simulink model "Full_Charge"  (R2020a)
settings: Solver=VariableStepAuto  StartTime=0.0  StopTime=45*60*60  RelTol=1e-3
values from neighbouring files (symbols this model uses):
  BlySyreON = 1    [sim_starter.m]
  CurrentChargeBlySyre = load    [sim_starter.m]
  CurrentChargeLiLille = load    [sim_starter.m]
  CurrentChargeLiStor = load    [sim_starter.m]
  CurrentChargeNiMH = load    [sim_starter.m]
  CurrentChargeSaltVand = load    [sim_starter.m]
  LiIonLilleON = 1    [sim_starter.m]
  LiIonStorON = 1    [sim_starter.m]
  NiMHON = 1    [sim_starter.m]
  SaltVandON = 1    [sim_starter.m]
  SwitchCurrentBlySyre = 1    [sim_starter.m]
  SwitchCurrentLiLille = 1    [sim_starter.m]
  SwitchCurrentLiStor = 1    [sim_starter.m]
  SwitchCurrentNiMH = 1    [sim_starter.m]
  SwitchCurrentSaltVand = 1    [sim_starter.m]
  VoltageChargeBlySyre = 0    [sim_starter.m]
  VoltageChargeLiLille = load    [sim_starter.m]
  VoltageChargeLiStor = load    [sim_starter.m]
  VoltageChargeNiMH = load    [sim_starter.m]
  VoltageChargeSaltVand = load    [sim_starter.m]
undefined symbols (not defined in the file or in its folder): Hydride, Metal, Nickel
libraries: nesl_utility x37, fl_lib x35, ee_lib x8, powerlib x7, electricdrivelib x1
(part 1 of 2)
settings Model: Creator=phili  LastModifiedBy=jenslawl

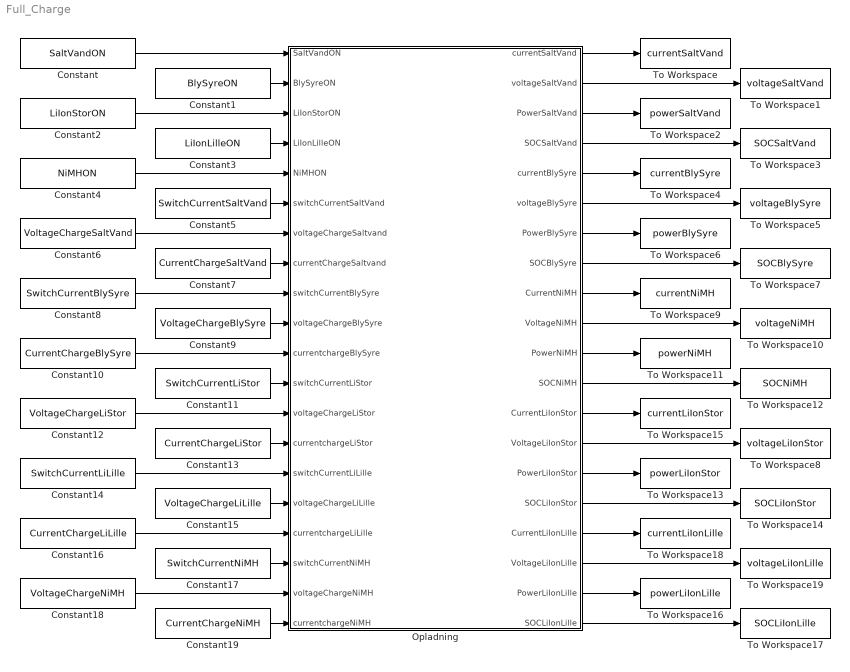
== system Full_Charge ==
  Constant : Constant  Value=SaltVandON
  Constant1 : Constant  Value=BlySyreON
  Constant10 : Constant  Value=CurrentChargeBlySyre
  Constant11 : Constant  Value=SwitchCurrentLiStor
  Constant12 : Constant  Value=VoltageChargeLiStor
  Constant13 : Constant  Value=CurrentChargeLiStor
  Constant14 : Constant  Value=SwitchCurrentLiLille
  Constant15 : Constant  Value=VoltageChargeLiLille
  Constant16 : Constant  Value=CurrentChargeLiLille
  Constant17 : Constant  Value=SwitchCurrentNiMH
  Constant18 : Constant  Value=VoltageChargeNiMH
  Constant19 : Constant  Value=CurrentChargeNiMH
  Constant2 : Constant  Value=LiIonStorON
  Constant3 : Constant  Value=LiIonLilleON
  Constant4 : Constant  Value=NiMHON
  Constant5 : Constant  Value=SwitchCurrentSaltVand
  Constant6 : Constant  Value=VoltageChargeSaltVand
  Constant7 : Constant  Value=CurrentChargeSaltVand
  Constant8 : Constant  Value=SwitchCurrentBlySyre
  Constant9 : Constant  Value=VoltageChargeBlySyre
  Opladning : Subsystem
  To Workspace : ToWorkspace  VariableName=currentSaltVand  SampleTime=-1
  To Workspace1 : ToWorkspace  VariableName=voltageSaltVand  SampleTime=-1
  To Workspace10 : ToWorkspace  VariableName=voltageNiMH  SampleTime=-1
  To Workspace11 : ToWorkspace  VariableName=powerNiMH  SampleTime=-1
  To Workspace12 : ToWorkspace  VariableName=SOCNiMH  SampleTime=-1
  To Workspace13 : ToWorkspace  VariableName=powerLiIonStor  SampleTime=-1
  To Workspace14 : ToWorkspace  VariableName=SOCLiIonStor  SampleTime=-1
  To Workspace15 : ToWorkspace  VariableName=currentLiIonStor  SampleTime=-1
  To Workspace16 : ToWorkspace  VariableName=powerLiIonLille  SampleTime=-1
  To Workspace17 : ToWorkspace  VariableName=SOCLiIonLille  SampleTime=-1
  To Workspace18 : ToWorkspace  VariableName=currentLiIonLille  SampleTime=-1
  To Workspace19 : ToWorkspace  VariableName=voltageLiIonLille  SampleTime=-1
  To Workspace2 : ToWorkspace  VariableName=powerSaltVand  SampleTime=-1
  To Workspace3 : ToWorkspace  VariableName=SOCSaltVand  SampleTime=-1
  To Workspace4 : ToWorkspace  VariableName=currentBlySyre  SampleTime=-1
  To Workspace5 : ToWorkspace  VariableName=voltageBlySyre  SampleTime=-1
  To Workspace6 : ToWorkspace  VariableName=powerBlySyre  SampleTime=-1
  To Workspace7 : ToWorkspace  VariableName=SOCBlySyre  SampleTime=-1
  To Workspace8 : ToWorkspace  VariableName=voltageLiIonStor  SampleTime=-1
  To Workspace9 : ToWorkspace  VariableName=currentNiMH  SampleTime=-1
  wires:
  Constant/1 -> Opladning/1(SaltVandON)
  Constant1/1 -> Opladning/2(BlySyreON)
  Constant2/1 -> Opladning/3(LiIonStorON)
  Constant3/1 -> Opladning/4(LiIonLilleON)
  Constant4/1 -> Opladning/5(NiMHON)
  Constant5/1 -> Opladning/6(switchCurrentSaltVand)
  Constant6/1 -> Opladning/7(voltageChargeSaltvand)
  Constant7/1 -> Opladning/8(currentChargeSaltvand)
  Constant8/1 -> Opladning/9(switchCurrentBlySyre)
  Constant9/1 -> Opladning/10(voltageChargeBlySyre)
  Constant10/1 -> Opladning/11(currentchargeBlySyre)
  Constant11/1 -> Opladning/12(switchCurrentLiStor)
  Constant12/1 -> Opladning/13(voltageChargeLiStor)
  Constant13/1 -> Opladning/14(currentchargeLiStor)
  Constant14/1 -> Opladning/15(switchCurrentLiLille)
  Constant15/1 -> Opladning/16(voltageChargeLiLille)
  Constant16/1 -> Opladning/17(currentchargeLiLille)
  Constant17/1 -> Opladning/18(switchCurrentNiMH)
  Constant18/1 -> Opladning/19(voltageChargeNiMH)
  Constant19/1 -> Opladning/20(currentchargeNiMH)
  Opladning/5(currentBlySyre) -> To Workspace4/1
  Opladning/12(SOCNiMH) -> To Workspace12/1
  Opladning/6(voltageBlySyre) -> To Workspace5/1
  Opladning/11(PowerNiMH) -> To Workspace11/1
  Opladning/8(SOCBlySyre) -> To Workspace7/1
  Opladning/13(CurrentLiIonStor) -> To Workspace15/1
  Opladning/7(PowerBlySyre) -> To Workspace6/1
  Opladning/4(SOCSaltVand) -> To Workspace3/1
  Opladning/18(VoltageLiIonLille) -> To Workspace19/1
  Opladning/2(voltageSaltVand) -> To Workspace1/1
  Opladning/3(PowerSaltVand) -> To Workspace2/1
  Opladning/20(SOCLiIonLille) -> To Workspace17/1
  Opladning/19(PowerLiIonLille) -> To Workspace16/1
  Opladning/9(CurrentNiMH) -> To Workspace9/1
  Opladning/14(VoltageLiIonStor) -> To Workspace8/1
  Opladning/15(PowerLiIonStor) -> To Workspace13/1
  Opladning/16(SOCLiIonStor) -> To Workspace14/1
  Opladning/10(VoltageNiMH) -> To Workspace10/1
  Opladning/1(currentSaltVand) -> To Workspace/1
  Opladning/17(CurrentLiIonLille) -> To Workspace18/1

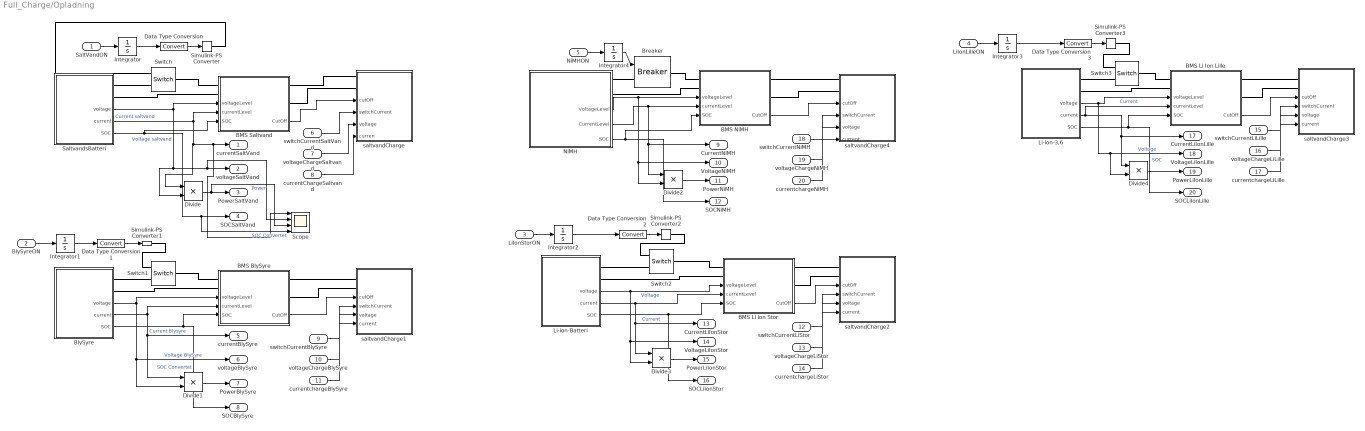
== system Full_Charge/Opladning ==
  SaltVandON : Inport
  BlySyreON : Inport  Port=2
  LiIonStorON : Inport  Port=3
  LiIonLilleON : Inport  Port=4
  NiMHON : Inport  Port=5
  switchCurrentSaltVand : Inport  Port=6
  voltageChargeSaltvand : Inport  Port=7
  currentChargeSaltvand : Inport  Port=8
  switchCurrentBlySyre : Inport  Port=9
  voltageChargeBlySyre : Inport  Port=10
  currentchargeBlySyre : Inport  Port=11
  switchCurrentLiStor : Inport  Port=12
  voltageChargeLiStor : Inport  Port=13
  currentchargeLiStor : Inport  Port=14
  switchCurrentLiLille : Inport  Port=15
  voltageChargeLiLille : Inport  Port=16
  currentchargeLiLille : Inport  Port=17
  switchCurrentNiMH : Inport  Port=18
  voltageChargeNiMH : Inport  Port=19
  currentchargeNiMH : Inport  Port=20
  BMS BlySyre : Subsystem
      settings: PortSchema="{\"entries\":[{\"content\":{\"sides\":[{\"content\":{\"connectorIds\":[\"LConn1\",\"LConn2\",\"In1\",\"In2\",\"In3\"]},\"type\":\"ConnectorPlacement.EquallySpacedRectSide\",\"uuid\":\"8e5b19d5-26fd-4308-a068-31d3a7110353\"},{\"content\":{\"connectorIds\":[\"RConn1\",\"RConn2\",\"Out1\"],\"side\":\"RIGHT\"},\"type\":\"ConnectorPlacement.EquallySpacedRectSide\",\"uuid\":\"43c00b24-a96d-45dd-baf7-73862471a89e\"},{\"content\":{\"connectorIds\":[],\"side\":\"TOP\"},\"type\":\"ConnectorPlacement.EquallySpacedRectSide\",\"uuid\":\"aec9a084-a9ff-4300-b99c-89bc23ebac6c\"}]},\"type\":\"ConnectorPlacement.EquallySpacedConnector\",\"uuid\":\"d767dd7e-ef5e-469c-820c-a4f5797d1fb9\"}],\"packageUris\":[\"http://schema.mathworks.com/mf0/Connector/19700101\"],\"version\":\"1.0\"}"
  BMS Li Ion Lille : Subsystem
      settings: PortSchema="{\"entries\":[{\"content\":{\"sides\":[{\"content\":{\"connectorIds\":[\"LConn1\",\"LConn2\",\"In1\",\"In2\",\"In3\"]},\"type\":\"ConnectorPlacement.EquallySpacedRectSide\",\"uuid\":\"8e5b19d5-26fd-4308-a068-31d3a7110353\"},{\"content\":{\"connectorIds\":[\"RConn1\",\"RConn2\",\"Out1\"],\"side\":\"RIGHT\"},\"type\":\"ConnectorPlacement.EquallySpacedRectSide\",\"uuid\":\"43c00b24-a96d-45dd-baf7-73862471a89e\"},{\"content\":{\"connectorIds\":[],\"side\":\"TOP\"},\"type\":\"ConnectorPlacement.EquallySpacedRectSide\",\"uuid\":\"aec9a084-a9ff-4300-b99c-89bc23ebac6c\"}]},\"type\":\"ConnectorPlacement.EquallySpacedConnector\",\"uuid\":\"d767dd7e-ef5e-469c-820c-a4f5797d1fb9\"}],\"packageUris\":[\"http://schema.mathworks.com/mf0/Connector/19700101\"],\"version\":\"1.0\"}"
  BMS Li ion Stor : Subsystem
      settings: PortSchema="{\"entries\":[{\"content\":{\"sides\":[{\"content\":{\"connectorIds\":[\"LConn1\",\"LConn2\",\"In1\",\"In2\",\"In3\"]},\"type\":\"ConnectorPlacement.EquallySpacedRectSide\",\"uuid\":\"8e5b19d5-26fd-4308-a068-31d3a7110353\"},{\"content\":{\"connectorIds\":[\"RConn1\",\"RConn2\",\"Out1\"],\"side\":\"RIGHT\"},\"type\":\"ConnectorPlacement.EquallySpacedRectSide\",\"uuid\":\"43c00b24-a96d-45dd-baf7-73862471a89e\"},{\"content\":{\"connectorIds\":[],\"side\":\"TOP\"},\"type\":\"ConnectorPlacement.EquallySpacedRectSide\",\"uuid\":\"aec9a084-a9ff-4300-b99c-89bc23ebac6c\"}]},\"type\":\"ConnectorPlacement.EquallySpacedConnector\",\"uuid\":\"d767dd7e-ef5e-469c-820c-a4f5797d1fb9\"}],\"packageUris\":[\"http://schema.mathworks.com/mf0/Connector/19700101\"],\"version\":\"1.0\"}"
  BMS NiMH : Subsystem
      settings: PortSchema="{\"entries\":[{\"content\":{\"sides\":[{\"content\":{\"connectorIds\":[\"LConn1\",\"LConn2\",\"In1\",\"In2\",\"In3\"]},\"type\":\"ConnectorPlacement.EquallySpacedRectSide\",\"uuid\":\"8e5b19d5-26fd-4308-a068-31d3a7110353\"},{\"content\":{\"connectorIds\":[\"RConn1\",\"RConn2\",\"Out1\"],\"side\":\"RIGHT\"},\"type\":\"ConnectorPlacement.EquallySpacedRectSide\",\"uuid\":\"43c00b24-a96d-45dd-baf7-73862471a89e\"},{\"content\":{\"connectorIds\":[],\"side\":\"TOP\"},\"type\":\"ConnectorPlacement.EquallySpacedRectSide\",\"uuid\":\"aec9a084-a9ff-4300-b99c-89bc23ebac6c\"}]},\"type\":\"ConnectorPlacement.EquallySpacedConnector\",\"uuid\":\"d767dd7e-ef5e-469c-820c-a4f5797d1fb9\"}],\"packageUris\":[\"http://schema.mathworks.com/mf0/Connector/19700101\"],\"version\":\"1.0\"}"
  "BMS Saltvand " : Subsystem
      settings: PortSchema="{\"entries\":[{\"content\":{\"sides\":[{\"content\":{\"connectorIds\":[\"LConn1\",\"LConn2\",\"In1\",\"In2\",\"In3\"]},\"type\":\"ConnectorPlacement.EquallySpacedRectSide\",\"uuid\":\"8e5b19d5-26fd-4308-a068-31d3a7110353\"},{\"content\":{\"connectorIds\":[\"RConn1\",\"RConn2\",\"Out1\"],\"side\":\"RIGHT\"},\"type\":\"ConnectorPlacement.EquallySpacedRectSide\",\"uuid\":\"43c00b24-a96d-45dd-baf7-73862471a89e\"},{\"content\":{\"connectorIds\":[],\"side\":\"TOP\"},\"type\":\"ConnectorPlacement.EquallySpacedRectSide\",\"uuid\":\"aec9a084-a9ff-4300-b99c-89bc23ebac6c\"}]},\"type\":\"ConnectorPlacement.EquallySpacedConnector\",\"uuid\":\"d767dd7e-ef5e-469c-820c-a4f5797d1fb9\"}],\"packageUris\":[\"http://schema.mathworks.com/mf0/Connector/19700101\"],\"version\":\"1.0\"}"
  BlySyre : Subsystem
      settings: PortSchema="{\"entries\":[{\"content\":{\"sides\":[{\"content\":{\"connectorIds\":[]},\"type\":\"ConnectorPlacement.EquallySpacedRectSide\",\"uuid\":\"b7adcffb-368c-467a-b339-3146d53f89f7\"},{\"content\":{\"connectorIds\":[\"RConn1\",\"RConn2\",\"Out1\",\"Out2\",\"Out3\"],\"side\":\"RIGHT\"},\"type\":\"ConnectorPlacement.EquallySpacedRectSide\",\"uuid\":\"78fa0dc6-8b86-442a-9e1f-c20c2cc39690\"},{\"content\":{\"connectorIds\":[],\"side\":\"TOP\"},\"type\":\"ConnectorPlacement.EquallySpacedRectSide\",\"uuid\":\"02b6bb54-52f8-4387-9821-90c0e82d6c22\"}]},\"type\":\"ConnectorPlacement.EquallySpacedConnector\",\"uuid\":\"f2eebdbf-49bd-409e-a7c0-76b4bde01873\"}],\"packageUris\":[\"http://schema.mathworks.com/mf0/Connector/19700101\"],\"version\":\"1.0\"}"
  Breaker : powerlib/Elements/Breaker  InitialState=0  SwitchingTimes="[1/60  5/60]"  External=on  BreakerResistance=0.01  SnubberResistance=1e6  SnubberCapacitance=inf  Measurements=None  MoreParameters=on  NoBreakLoop=off
  Data Type Conversion{,1..3} (4 alike) : DataTypeConversion
  Divide{,1..4} (5 alike) : Product  Inputs=**
  Integrator{,1..4} (5 alike) : Integrator
  Li-ion-3,6 : Subsystem
      settings: PortSchema="{\"entries\":[{\"content\":{\"sides\":[{\"content\":{\"connectorIds\":[]},\"type\":\"ConnectorPlacement.EquallySpacedRectSide\",\"uuid\":\"b7adcffb-368c-467a-b339-3146d53f89f7\"},{\"content\":{\"connectorIds\":[\"RConn1\",\"RConn2\",\"Out1\",\"Out2\",\"Out3\"],\"side\":\"RIGHT\"},\"type\":\"ConnectorPlacement.EquallySpacedRectSide\",\"uuid\":\"78fa0dc6-8b86-442a-9e1f-c20c2cc39690\"},{\"content\":{\"connectorIds\":[],\"side\":\"TOP\"},\"type\":\"ConnectorPlacement.EquallySpacedRectSide\",\"uuid\":\"02b6bb54-52f8-4387-9821-90c0e82d6c22\"}]},\"type\":\"ConnectorPlacement.EquallySpacedConnector\",\"uuid\":\"f2eebdbf-49bd-409e-a7c0-76b4bde01873\"}],\"packageUris\":[\"http://schema.mathworks.com/mf0/Connector/19700101\"],\"version\":\"1.0\"}"
  Li-ion-Batteri : Subsystem
      settings: PortSchema="{\"entries\":[{\"content\":{\"sides\":[{\"content\":{\"connectorIds\":[]},\"type\":\"ConnectorPlacement.EquallySpacedRectSide\",\"uuid\":\"b7adcffb-368c-467a-b339-3146d53f89f7\"},{\"content\":{\"connectorIds\":[\"RConn1\",\"RConn2\",\"Out1\",\"Out2\",\"Out3\"],\"side\":\"RIGHT\"},\"type\":\"ConnectorPlacement.EquallySpacedRectSide\",\"uuid\":\"78fa0dc6-8b86-442a-9e1f-c20c2cc39690\"},{\"content\":{\"connectorIds\":[],\"side\":\"TOP\"},\"type\":\"ConnectorPlacement.EquallySpacedRectSide\",\"uuid\":\"02b6bb54-52f8-4387-9821-90c0e82d6c22\"}]},\"type\":\"ConnectorPlacement.EquallySpacedConnector\",\"uuid\":\"f2eebdbf-49bd-409e-a7c0-76b4bde01873\"}],\"packageUris\":[\"http://schema.mathworks.com/mf0/Connector/19700101\"],\"version\":\"1.0\"}"
  NiMH : Subsystem
      settings: PortSchema="{\"entries\":[{\"content\":{\"sides\":[{\"content\":{\"connectorIds\":[]},\"type\":\"ConnectorPlacement.EquallySpacedRectSide\",\"uuid\":\"fc65cf16-1b08-48cf-a4b8-6124313288b7\"},{\"content\":{\"connectorIds\":[\"RConn1\",\"RConn2\",\"Out1\",\"Out2\",\"Out3\"],\"side\":\"RIGHT\"},\"type\":\"ConnectorPlacement.EquallySpacedRectSide\",\"uuid\":\"2587f880-824f-409e-889d-6e6395f8efa4\"},{\"content\":{\"connectorIds\":[],\"side\":\"TOP\"},\"type\":\"ConnectorPlacement.EquallySpacedRectSide\",\"uuid\":\"a61b6a50-66af-4684-a024-cf79c14250f1\"}]},\"type\":\"ConnectorPlacement.EquallySpacedConnector\",\"uuid\":\"60ef1120-39c0-433f-916b-5d1a9aec7516\"}],\"packageUris\":[\"http://schema.mathworks.com/mf0/Connector/19700101\"],\"version\":\"1.0\"}"
  SaltvandsBatteri : Subsystem
      settings: PortSchema="{\"entries\":[{\"content\":{\"sides\":[{\"content\":{\"connectorIds\":[]},\"type\":\"ConnectorPlacement.EquallySpacedRectSide\",\"uuid\":\"b7adcffb-368c-467a-b339-3146d53f89f7\"},{\"content\":{\"connectorIds\":[\"RConn1\",\"RConn2\",\"Out1\",\"Out2\",\"Out3\"],\"side\":\"RIGHT\"},\"type\":\"ConnectorPlacement.EquallySpacedRectSide\",\"uuid\":\"78fa0dc6-8b86-442a-9e1f-c20c2cc39690\"},{\"content\":{\"connectorIds\":[],\"side\":\"TOP\"},\"type\":\"ConnectorPlacement.EquallySpacedRectSide\",\"uuid\":\"02b6bb54-52f8-4387-9821-90c0e82d6c22\"}]},\"type\":\"ConnectorPlacement.EquallySpacedConnector\",\"uuid\":\"f2eebdbf-49bd-409e-a7c0-76b4bde01873\"}],\"packageUris\":[\"http://schema.mathworks.com/mf0/Connector/19700101\"],\"version\":\"1.0\"}"
  Scope : Scope  NumInputPorts=4
  Simulink-PS Converter{,1..3} (4 alike) : nesl_utility/Simulink-PS Converter  PhysicalDomain=network_engine_domain  SubClassName=ps_input  LeftPortType=input  RightPortType=output  PseudoPeriodic=off  Frequencies=[]  NoiseDistribution=none  NoiseParameters=[]  Unit=V  AffineConversion=on  FilteringAndDerivatives=provide  SimscapeFilterOrder=1  InputFilterTimeConstant=0.001  UdotUserProvided=0
  Switch{,1..3} (4 alike) : fl_lib/Electrical/Electrical Elements/Switch  R_closed=0.01 Ohm  G_open=1e-8 1/Ohm  Threshold=0.5  i_specify=off  i_priority=None  i=0 A  i_nominal_specify=off  i_nominal_unit=A  i_nominal_value=1  v_specify=off  v_priority=None  v=0 V  v_nominal_specify=off  v_nominal_unit=V  v_nominal_value=1
  saltvandCharge : Subsystem
      settings: PortSchema="{\"entries\":[{\"content\":{\"sides\":[{\"content\":{\"connectorIds\":[\"LConn1\",\"LConn2\",\"In1\",\"In2\",\"In3\",\"In4\"]},\"type\":\"ConnectorPlacement.EquallySpacedRectSide\",\"uuid\":\"2e353d4e-3f49-4579-a255-425bfce684d6\"},{\"content\":{\"connectorIds\":[],\"side\":\"RIGHT\"},\"type\":\"ConnectorPlacement.EquallySpacedRectSide\",\"uuid\":\"34cbc265-6c91-4c9c-8158-5747a5c43dbf\"},{\"content\":{\"connectorIds\":[],\"side\":\"TOP\"},\"type\":\"ConnectorPlacement.EquallySpacedRectSide\",\"uuid\":\"50fae68b-9589-49f5-b407-e6af6c9daf90\"}]},\"type\":\"ConnectorPlacement.EquallySpacedConnector\",\"uuid\":\"570e30f3-d8b6-4d6b-9284-8ec4f252a65f\"}],\"packageUris\":[\"http://schema.mathworks.com/mf0/Connector/19700101\"],\"version\":\"1.0\"}"
  saltvandCharge1 : Subsystem
      settings: PortSchema="{\"entries\":[{\"content\":{\"sides\":[{\"content\":{\"connectorIds\":[\"LConn1\",\"LConn2\",\"In1\",\"In2\",\"In3\",\"In4\"]},\"type\":\"ConnectorPlacement.EquallySpacedRectSide\",\"uuid\":\"e7e8623b-c175-48fc-95e1-1b985925c164\"},{\"content\":{\"connectorIds\":[],\"side\":\"RIGHT\"},\"type\":\"ConnectorPlacement.EquallySpacedRectSide\",\"uuid\":\"0543124e-c3bb-4fd2-8f85-0af0b394bb91\"},{\"content\":{\"connectorIds\":[],\"side\":\"TOP\"},\"type\":\"ConnectorPlacement.EquallySpacedRectSide\",\"uuid\":\"9e5814f1-686b-4368-be8f-3ed792b49e24\"}]},\"type\":\"ConnectorPlacement.EquallySpacedConnector\",\"uuid\":\"44836dfd-9a6b-4a07-8653-d78a378bec5b\"}],\"packageUris\":[\"http://schema.mathworks.com/mf0/Connector/19700101\"],\"version\":\"1.0\"}"
  saltvandCharge2 : Subsystem
      settings: PortSchema="{\"entries\":[{\"content\":{\"sides\":[{\"content\":{\"connectorIds\":[\"LConn1\",\"LConn2\",\"In1\",\"In2\",\"In3\",\"In4\"]},\"type\":\"ConnectorPlacement.EquallySpacedRectSide\",\"uuid\":\"e7e8623b-c175-48fc-95e1-1b985925c164\"},{\"content\":{\"connectorIds\":[],\"side\":\"RIGHT\"},\"type\":\"ConnectorPlacement.EquallySpacedRectSide\",\"uuid\":\"0543124e-c3bb-4fd2-8f85-0af0b394bb91\"},{\"content\":{\"connectorIds\":[],\"side\":\"TOP\"},\"type\":\"ConnectorPlacement.EquallySpacedRectSide\",\"uuid\":\"9e5814f1-686b-4368-be8f-3ed792b49e24\"}]},\"type\":\"ConnectorPlacement.EquallySpacedConnector\",\"uuid\":\"44836dfd-9a6b-4a07-8653-d78a378bec5b\"}],\"packageUris\":[\"http://schema.mathworks.com/mf0/Connector/19700101\"],\"version\":\"1.0\"}"
  saltvandCharge3 : Subsystem
      settings: PortSchema="{\"entries\":[{\"content\":{\"sides\":[{\"content\":{\"connectorIds\":[\"LConn1\",\"LConn2\",\"In1\",\"In2\",\"In3\",\"In4\"]},\"type\":\"ConnectorPlacement.EquallySpacedRectSide\",\"uuid\":\"e7e8623b-c175-48fc-95e1-1b985925c164\"},{\"content\":{\"connectorIds\":[],\"side\":\"RIGHT\"},\"type\":\"ConnectorPlacement.EquallySpacedRectSide\",\"uuid\":\"0543124e-c3bb-4fd2-8f85-0af0b394bb91\"},{\"content\":{\"connectorIds\":[],\"side\":\"TOP\"},\"type\":\"ConnectorPlacement.EquallySpacedRectSide\",\"uuid\":\"9e5814f1-686b-4368-be8f-3ed792b49e24\"}]},\"type\":\"ConnectorPlacement.EquallySpacedConnector\",\"uuid\":\"44836dfd-9a6b-4a07-8653-d78a378bec5b\"}],\"packageUris\":[\"http://schema.mathworks.com/mf0/Connector/19700101\"],\"version\":\"1.0\"}"
  saltvandCharge4 : Subsystem
      settings: PortSchema="{\"entries\":[{\"content\":{\"sides\":[{\"content\":{\"connectorIds\":[\"LConn1\",\"LConn2\",\"In1\",\"In2\",\"In3\",\"In4\"]},\"type\":\"ConnectorPlacement.EquallySpacedRectSide\",\"uuid\":\"e7e8623b-c175-48fc-95e1-1b985925c164\"},{\"content\":{\"connectorIds\":[],\"side\":\"RIGHT\"},\"type\":\"ConnectorPlacement.EquallySpacedRectSide\",\"uuid\":\"0543124e-c3bb-4fd2-8f85-0af0b394bb91\"},{\"content\":{\"connectorIds\":[],\"side\":\"TOP\"},\"type\":\"ConnectorPlacement.EquallySpacedRectSide\",\"uuid\":\"9e5814f1-686b-4368-be8f-3ed792b49e24\"}]},\"type\":\"ConnectorPlacement.EquallySpacedConnector\",\"uuid\":\"44836dfd-9a6b-4a07-8653-d78a378bec5b\"}],\"packageUris\":[\"http://schema.mathworks.com/mf0/Connector/19700101\"],\"version\":\"1.0\"}"
  currentSaltVand : Outport
  voltageSaltVand : Outport  Port=2
  PowerSaltVand : Outport  Port=3
  SOCSaltVand : Outport  Port=4
  currentBlySyre : Outport  Port=5
  voltageBlySyre : Outport  Port=6
  PowerBlySyre : Outport  Port=7
  SOCBlySyre : Outport  Port=8
  CurrentNiMH : Outport  Port=9
  VoltageNiMH : Outport  Port=10
  PowerNiMH : Outport  Port=11
  SOCNiMH : Outport  Port=12
  CurrentLiIonStor : Outport  Port=13
  VoltageLiIonStor : Outport  Port=14
  PowerLiIonStor : Outport  Port=15
  SOCLiIonStor : Outport  Port=16
  CurrentLiIonLille : Outport  Port=17
  VoltageLiIonLille : Outport  Port=18
  PowerLiIonLille : Outport  Port=19
  SOCLiIonLille : Outport  Port=20
  wires:
  voltageChargeNiMH/1 -> saltvandCharge4/3(voltage)
  SaltvandsBatteri/2(current) -> Scope/1, currentSaltVand/1, Divide/1, "BMS Saltvand "/2(currentLevel)  "Current saltvand"
  Integrator1/1 -> Data Type Conversion1/1
  Data Type Conversion2/1 -> Simulink-PS Converter2/1
  Integrator3/1 -> Data Type Conversion3/1
  Li-ion-3,6/1(voltage) -> BMS Li Ion Lille/1(voltageLevel), VoltageLiIonLille/1, Divide4/2  "Voltage"
  Divide1/1 -> PowerBlySyre/1
  Data Type Conversion1/1 -> Simulink-PS Converter1/1
  Divide/1 -> Scope/3, PowerSaltVand/1  "Power"
  Li-ion-3,6/3(SOC) -> SOCLiIonLille/1, BMS Li Ion Lille/3(SOC)  "SOC"
  NiMH/1(VoltageLevel) -> VoltageNiMH/1, Divide2/2, BMS NiMH/1(voltageLevel)
  NiMH/2(CurrentLevel) -> BMS NiMH/2(currentLevel), CurrentNiMH/1, Divide2/1
  Li-ion-Batteri/3(SOC) -> SOCLiIonStor/1, BMS Li ion Stor/3(SOC)
  Li-ion-Batteri/2(current) -> CurrentLiIonStor/1, Divide3/1, BMS Li ion Stor/2(currentLevel)  "Current"
  BlySyre/2(current) -> currentBlySyre/1, Divide1/1, BMS BlySyre/2(currentLevel)  "Current Blysyre"
  BlySyre/1(voltage) -> BMS BlySyre/1(voltageLevel), voltageBlySyre/1, Divide1/2  "Voltage BlySyre"
  BlySyre/3(SOC) -> SOCBlySyre/1, BMS BlySyre/3(SOC)  "SOC Convertet"
  BMS BlySyre/1(CutOff) -> saltvandCharge1/1(cutOff)
  SaltvandsBatteri/1(voltage) -> Scope/2, voltageSaltVand/1, Divide/2, "BMS Saltvand "/1(voltageLevel)  "Voltage saltvand"
  LiIonStorON/1 -> Integrator2/1
  Li-ion-3,6/2(current) -> CurrentLiIonLille/1, Divide4/1, BMS Li Ion Lille/2(currentLevel)  "Current"
  NiMH/3(SOC) -> SOCNiMH/1, BMS NiMH/3(SOC)
  SaltvandsBatteri/3(SOC) -> Scope/4, SOCSaltVand/1, "BMS Saltvand "/3(SOC)  "SOC Convertet"
  Divide4/1 -> PowerLiIonLille/1
  Data Type Conversion3/1 -> Simulink-PS Converter3/1
  switchCurrentNiMH/1 -> saltvandCharge4/2(switchCurrent)
  Data Type Conversion/1 -> Simulink-PS Converter/1
  Integrator2/1 -> Data Type Conversion2/1
  Li-ion-Batteri/1(voltage) -> VoltageLiIonStor/1, Divide3/2, BMS Li ion Stor/1(voltageLevel)  "Voltage"
  Integrator4/1 -> Breaker/1
  "BMS Saltvand "/1(CutOff) -> saltvandCharge/1(cutOff)
  Divide3/1 -> PowerLiIonStor/1
  switchCurrentLiStor/1 -> saltvandCharge2/2(switchCurrent)
  switchCurrentLiLille/1 -> saltvandCharge3/2(switchCurrent)
  LiIonLilleON/1 -> Integrator3/1
  BlySyreON/1 -> Integrator1/1
  NiMHON/1 -> Integrator4/1
  Divide2/1 -> PowerNiMH/1
  currentchargeNiMH/1 -> saltvandCharge4/4(current)
  Integrator/1 -> Data Type Conversion/1
  voltageChargeLiStor/1 -> saltvandCharge2/3(voltage)
  currentchargeLiStor/1 -> saltvandCharge2/4(current)
  BMS Li Ion Lille/1(CutOff) -> saltvandCharge3/1(cutOff)
  voltageChargeLiLille/1 -> saltvandCharge3/3(voltage)
  currentchargeLiLille/1 -> saltvandCharge3/4(current)
  BMS NiMH/1(CutOff) -> saltvandCharge4/1(cutOff)
  currentchargeBlySyre/1 -> saltvandCharge1/4(current)
  voltageChargeBlySyre/1 -> saltvandCharge1/3(voltage)
  switchCurrentBlySyre/1 -> saltvandCharge1/2(switchCurrent)
  BMS Li ion Stor/1(CutOff) -> saltvandCharge2/1(cutOff)
  SaltVandON/1 -> Integrator/1
  switchCurrentSaltVand/1 -> saltvandCharge/2(switchCurrent)
  voltageChargeSaltvand/1 -> saltvandCharge/3(voltage)
  currentChargeSaltvand/1 -> saltvandCharge/4(curren)
  connections:
  BlySyre/RConn2 -- BMS BlySyre/LConn2
  Simulink-PS Converter/RConn1 -- Switch/RConn1
  BMS NiMH/RConn1 -- saltvandCharge4/LConn1
  BMS Li ion Stor/RConn1 -- saltvandCharge2/LConn1
  SaltvandsBatteri/RConn2 -- "BMS Saltvand "/LConn2
  Switch1/RConn2 -- BlySyre/RConn1
  Simulink-PS Converter1/RConn1 -- Switch1/RConn1
  Li-ion-3,6/RConn2 -- BMS Li Ion Lille/LConn2
  Li-ion-Batteri/RConn1 -- Switch2/RConn2
  BMS Li ion Stor/LConn2 -- Li-ion-Batteri/RConn2
  Switch/LConn1 -- "BMS Saltvand "/LConn1
  NiMH/RConn2 -- BMS NiMH/LConn2
  Switch3/LConn1 -- BMS Li Ion Lille/LConn1
  Switch2/LConn1 -- BMS Li ion Stor/LConn1
  Simulink-PS Converter2/RConn1 -- Switch2/RConn1
  Simulink-PS Converter3/RConn1 -- Switch3/RConn1
  saltvandCharge3/LConn2 -- BMS Li Ion Lille/RConn2
  BMS Li ion Stor/RConn2 -- saltvandCharge2/LConn2
  Breaker/LConn1 -- NiMH/RConn1
  Switch/RConn2 -- SaltvandsBatteri/RConn1
  Breaker/RConn1 -- BMS NiMH/LConn1
  Switch3/RConn2 -- Li-ion-3,6/RConn1
  Switch1/LConn1 -- BMS BlySyre/LConn1
  BMS NiMH/RConn2 -- saltvandCharge4/LConn2
  saltvandCharge3/LConn1 -- BMS Li Ion Lille/RConn1
  saltvandCharge1/LConn1 -- BMS BlySyre/RConn1
  "BMS Saltvand "/RConn1 -- saltvandCharge/LConn1
  BMS BlySyre/RConn2 -- saltvandCharge1/LConn2
  "BMS Saltvand "/RConn2 -- saltvandCharge/LConn2

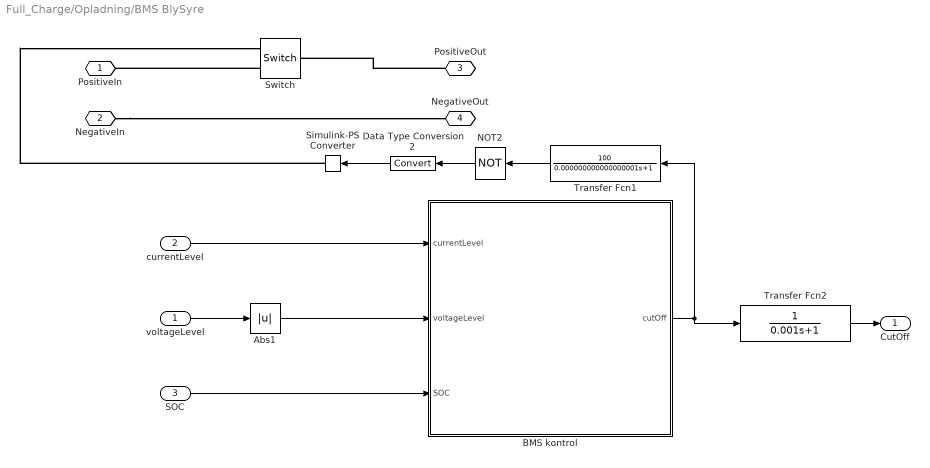
== system Full_Charge/Opladning/BMS BlySyre ==
  voltageLevel : Inport
  currentLevel : Inport  Port=2
  SOC : Inport  Port=3
  Abs1 : Abs
  BMS kontrol : Stateflow chart  TreatAsAtomicUnit=on
  Data Type Conversion2 : DataTypeConversion
  NOT2 : Logic  Operator=NOT  IconShape=distinctive  AllPortsSameDT=off  OutDataTypeStr=boolean
  Simulink-PS Converter : nesl_utility/Simulink-PS Converter  PhysicalDomain=network_engine_domain  SubClassName=ps_input  LeftPortType=input  RightPortType=output  PseudoPeriodic=off  Frequencies=[]  NoiseDistribution=none  NoiseParameters=[]  Unit=V  AffineConversion=off  FilteringAndDerivatives=provide  SimscapeFilterOrder=1  InputFilterTimeConstant=0.001  UdotUserProvided=0
  Switch : fl_lib/Electrical/Electrical Elements/Switch  R_closed=0.01 Ohm  G_open=1e-8 1/Ohm  Threshold=0.5  i_specify=off  i_priority=None  i=0 A  i_nominal_specify=off  i_nominal_unit=A  i_nominal_value=1  v_specify=off  v_priority=None  v=0 V  v_nominal_specify=off  v_nominal_unit=V  v_nominal_value=1
  Transfer Fcn1 : TransferFcn  Numerator=[100]  Denominator=[0.000000000000000001 1]
  Transfer Fcn2 : TransferFcn  Denominator=[0.001 1]
  PositiveIn : PMIOPort  Side=Left
  NegativeIn : PMIOPort  Port=2  Side=Left
  PositiveOut : PMIOPort  Port=3  Side=Right
  NegativeOut : PMIOPort  Port=4  Side=Right
  CutOff : Outport
  wires:
  SOC/1 -> BMS kontrol/3(SOC)
  BMS kontrol/1(cutOff) -> Transfer Fcn2/1, Transfer Fcn1/1
  currentLevel/1 -> BMS kontrol/1(currentLevel)
  voltageLevel/1 -> Abs1/1
  Transfer Fcn2/1 -> CutOff/1
  Abs1/1 -> BMS kontrol/2(voltageLevel)
  NOT2/1 -> Data Type Conversion2/1
  Transfer Fcn1/1 -> NOT2/1
  Data Type Conversion2/1 -> Simulink-PS Converter/1
  connections:
  NegativeIn/RConn1 -- NegativeOut/RConn1
  Switch/RConn2 -- PositiveIn/RConn1
  Simulink-PS Converter/RConn1 -- Switch/RConn1
  PositiveOut/RConn1 -- Switch/LConn1

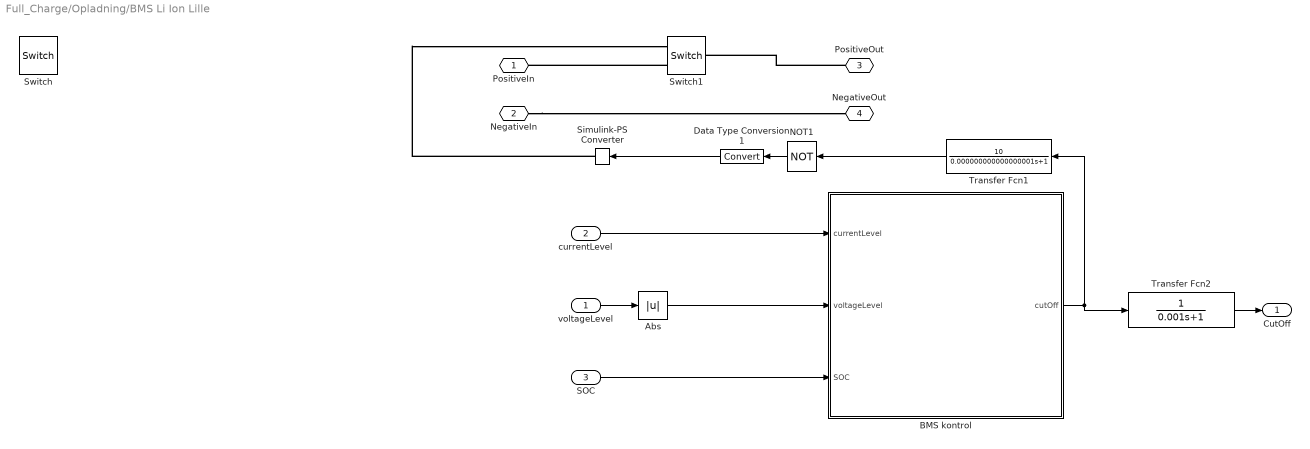
== system Full_Charge/Opladning/BMS Li Ion Lille ==
  voltageLevel : Inport
  currentLevel : Inport  Port=2
  SOC : Inport  Port=3
  Abs : Abs
  BMS kontrol : Stateflow chart  TreatAsAtomicUnit=on
  Data Type Conversion1 : DataTypeConversion
  NOT1 : Logic  Operator=NOT  IconShape=distinctive  AllPortsSameDT=off  OutDataTypeStr=boolean
  Simulink-PS Converter : nesl_utility/Simulink-PS Converter  PhysicalDomain=network_engine_domain  SubClassName=ps_input  LeftPortType=input  RightPortType=output  PseudoPeriodic=off  Frequencies=[]  NoiseDistribution=none  NoiseParameters=[]  Unit=V  AffineConversion=off  FilteringAndDerivatives=provide  SimscapeFilterOrder=1  InputFilterTimeConstant=0.001  UdotUserProvided=0
  Switch : fl_lib/Electrical/Electrical Elements/Switch  R_closed=0.01 Ohm  G_open=1e-8 1/Ohm  Threshold=0.5  i_specify=off  i_priority=None  i=0 A  i_nominal_specify=off  i_nominal_unit=A  i_nominal_value=1  v_specify=off  v_priority=None  v=0 V  v_nominal_specify=off  v_nominal_unit=V  v_nominal_value=1
  Switch1 : fl_lib/Electrical/Electrical Elements/Switch  R_closed=0.01 Ohm  G_open=1e-8 1/Ohm  Threshold=0.5  i_specify=off  i_priority=None  i=0 A  i_nominal_specify=off  i_nominal_unit=A  i_nominal_value=1  v_specify=off  v_priority=None  v=0 V  v_nominal_specify=off  v_nominal_unit=V  v_nominal_value=1
  Transfer Fcn1 : TransferFcn  Numerator=[10]  Denominator=[0.000000000000000001 1]
  Transfer Fcn2 : TransferFcn  Denominator=[0.001 1]
  PositiveIn : PMIOPort  Side=Left
  NegativeIn : PMIOPort  Port=2  Side=Left
  PositiveOut : PMIOPort  Port=3  Side=Right
  NegativeOut : PMIOPort  Port=4  Side=Right
  CutOff : Outport
  wires:
  Transfer Fcn2/1 -> CutOff/1
  voltageLevel/1 -> Abs/1
  currentLevel/1 -> BMS kontrol/1(currentLevel)
  BMS kontrol/1(cutOff) -> Transfer Fcn1/1, Transfer Fcn2/1
  SOC/1 -> BMS kontrol/3(SOC)
  Abs/1 -> BMS kontrol/2(voltageLevel)
  NOT1/1 -> Data Type Conversion1/1
  Data Type Conversion1/1 -> Simulink-PS Converter/1
  Transfer Fcn1/1 -> NOT1/1
  connections:
  PositiveOut/RConn1 -- Switch1/LConn1
  Simulink-PS Converter/RConn1 -- Switch1/RConn1
  Switch1/RConn2 -- PositiveIn/RConn1
  NegativeIn/RConn1 -- NegativeOut/RConn1

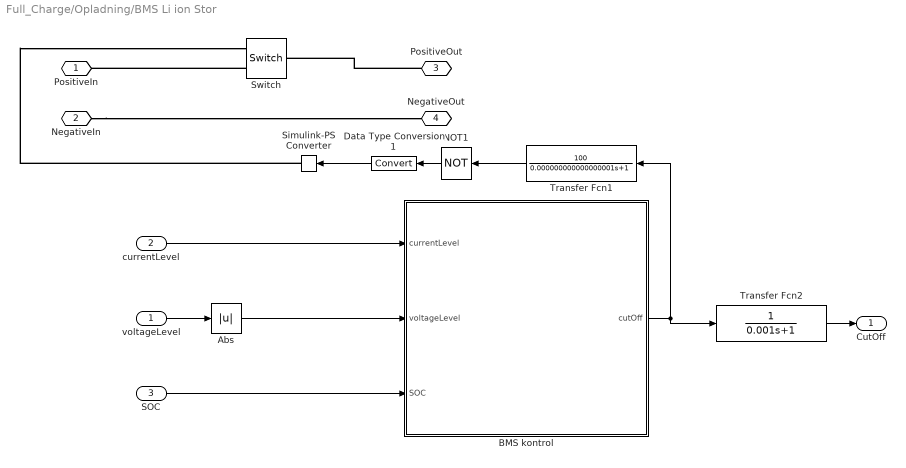
== system Full_Charge/Opladning/BMS Li ion Stor ==
  voltageLevel : Inport
  currentLevel : Inport  Port=2
  SOC : Inport  Port=3
  Abs : Abs
  BMS kontrol : Stateflow chart  TreatAsAtomicUnit=on
  Data Type Conversion1 : DataTypeConversion
  NOT1 : Logic  Operator=NOT  IconShape=distinctive  AllPortsSameDT=off  OutDataTypeStr=boolean
  Simulink-PS Converter : nesl_utility/Simulink-PS Converter  PhysicalDomain=network_engine_domain  SubClassName=ps_input  LeftPortType=input  RightPortType=output  PseudoPeriodic=off  Frequencies=[]  NoiseDistribution=none  NoiseParameters=[]  Unit=V  AffineConversion=off  FilteringAndDerivatives=provide  SimscapeFilterOrder=1  InputFilterTimeConstant=0.001  UdotUserProvided=0
  Switch : fl_lib/Electrical/Electrical Elements/Switch  R_closed=0.01 Ohm  G_open=1e-8 1/Ohm  Threshold=0.5  i_specify=off  i_priority=None  i=0 A  i_nominal_specify=off  i_nominal_unit=A  i_nominal_value=1  v_specify=off  v_priority=None  v=0 V  v_nominal_specify=off  v_nominal_unit=V  v_nominal_value=1
  Transfer Fcn1 : TransferFcn  Numerator=[100]  Denominator=[0.000000000000000001 1]
  Transfer Fcn2 : TransferFcn  Denominator=[0.001 1]
  PositiveIn : PMIOPort  Side=Left
  NegativeIn : PMIOPort  Port=2  Side=Left
  PositiveOut : PMIOPort  Port=3  Side=Right
  NegativeOut : PMIOPort  Port=4  Side=Right
  CutOff : Outport
  wires:
  Transfer Fcn2/1 -> CutOff/1
  voltageLevel/1 -> Abs/1
  currentLevel/1 -> BMS kontrol/1(currentLevel)
  BMS kontrol/1(cutOff) -> Transfer Fcn1/1, Transfer Fcn2/1
  SOC/1 -> BMS kontrol/3(SOC)
  Abs/1 -> BMS kontrol/2(voltageLevel)
  NOT1/1 -> Data Type Conversion1/1
  Transfer Fcn1/1 -> NOT1/1
  Data Type Conversion1/1 -> Simulink-PS Converter/1
  connections:
  PositiveOut/RConn1 -- Switch/LConn1
  Simulink-PS Converter/RConn1 -- Switch/RConn1
  Switch/RConn2 -- PositiveIn/RConn1
  NegativeIn/RConn1 -- NegativeOut/RConn1

== system Full_Charge/Opladning/BMS NiMH ==
  voltageLevel : Inport
  currentLevel : Inport  Port=2
  SOC : Inport  Port=3
  Abs : Abs
  BMS kontrol : Stateflow chart  TreatAsAtomicUnit=on
  Breaker : powerlib/Elements/Breaker  InitialState=1  SwitchingTimes="[1/60  5/60]"  External=on  BreakerResistance=0.01  SnubberResistance=1e6  SnubberCapacitance=inf  Measurements=None  MoreParameters=on  NoBreakLoop=off
  Transfer Fcn1 : TransferFcn  Numerator=[10]  Denominator=[0.000000000000000001 1]
  Transfer Fcn2 : TransferFcn  Denominator=[0.001 1]
  PositiveIn : PMIOPort  Side=Left
  NegativeIn : PMIOPort  Port=2  Side=Left
  PositiveOut : PMIOPort  Port=3  Side=Right
  NegativeOut : PMIOPort  Port=4  Side=Right
  CutOff : Outport
  wires:
  Transfer Fcn2/1 -> CutOff/1
  Transfer Fcn1/1 -> Breaker/1
  voltageLevel/1 -> Abs/1
  currentLevel/1 -> BMS kontrol/1(currentLevel)
  BMS kontrol/1(cutOff) -> Transfer Fcn1/1, Transfer Fcn2/1
  SOC/1 -> BMS kontrol/3(SOC)
  Abs/1 -> BMS kontrol/2(voltageLevel)
  connections:
  NegativeIn/RConn1 -- NegativeOut/RConn1
  Breaker/LConn1 -- PositiveIn/RConn1
  Breaker/RConn1 -- PositiveOut/RConn1

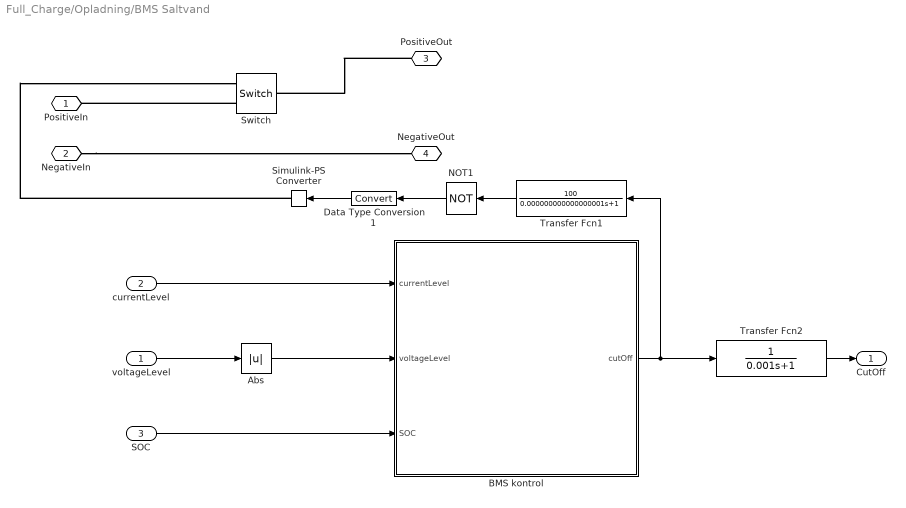
== system Full_Charge/Opladning/BMS Saltvand  ==
  voltageLevel : Inport
  currentLevel : Inport  Port=2
  SOC : Inport  Port=3
  Abs : Abs
  BMS kontrol : Stateflow chart  TreatAsAtomicUnit=on
  Data Type Conversion1 : DataTypeConversion
  NOT1 : Logic  Operator=NOT  IconShape=distinctive  AllPortsSameDT=off  OutDataTypeStr=boolean
  Simulink-PS Converter : nesl_utility/Simulink-PS Converter  PhysicalDomain=network_engine_domain  SubClassName=ps_input  LeftPortType=input  RightPortType=output  PseudoPeriodic=off  Frequencies=[]  NoiseDistribution=none  NoiseParameters=[]  Unit=V  AffineConversion=off  FilteringAndDerivatives=provide  SimscapeFilterOrder=1  InputFilterTimeConstant=0.001  UdotUserProvided=0
  Switch : fl_lib/Electrical/Electrical Elements/Switch  R_closed=0.01 Ohm  G_open=1e-8 1/Ohm  Threshold=0.5  i_specify=off  i_priority=None  i=0 A  i_nominal_specify=off  i_nominal_unit=A  i_nominal_value=1  v_specify=off  v_priority=None  v=0 V  v_nominal_specify=off  v_nominal_unit=V  v_nominal_value=1
  Transfer Fcn1 : TransferFcn  Numerator=[100]  Denominator=[0.000000000000000001 1]
  Transfer Fcn2 : TransferFcn  Denominator=[0.001 1]
  PositiveIn : PMIOPort  Side=Left
  NegativeIn : PMIOPort  Port=2  Side=Left
  PositiveOut : PMIOPort  Port=3  Side=Right
  NegativeOut : PMIOPort  Port=4  Side=Right
  CutOff : Outport
  wires:
  SOC/1 -> BMS kontrol/3(SOC)
  BMS kontrol/1(cutOff) -> Transfer Fcn1/1, Transfer Fcn2/1
  currentLevel/1 -> BMS kontrol/1(currentLevel)
  voltageLevel/1 -> Abs/1
  Transfer Fcn2/1 -> CutOff/1
  Abs/1 -> BMS kontrol/2(voltageLevel)
  NOT1/1 -> Data Type Conversion1/1
  Data Type Conversion1/1 -> Simulink-PS Converter/1
  Transfer Fcn1/1 -> NOT1/1
  connections:
  NegativeIn/RConn1 -- NegativeOut/RConn1
  Switch/RConn2 -- PositiveIn/RConn1
  Simulink-PS Converter/RConn1 -- Switch/RConn1
  PositiveOut/RConn1 -- Switch/LConn1

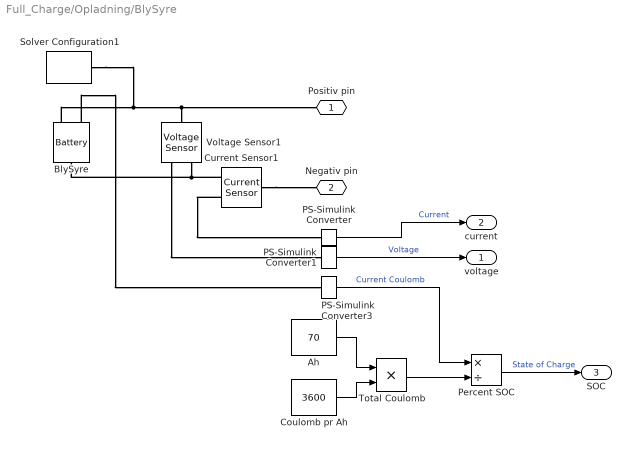
== system Full_Charge/Opladning/BlySyre ==
  Ah : Constant  Value=70
  BlySyre : ee_lib/Sources/Battery  Vnom=12 V  R1=0.001 Ohm  prm_AH=2  AH=70 hr*A  V1=10.8 V  AH1=35 hr*A  prm_R2=2  R2=2.47 kOhm  prm_dyn=2  Rp1=0.0007 Ohm  tau1=5000 s  Rp2=0.007 Ohm  tau2=50 s  Rp3=0.005 Ohm  tau3=30 s  Rp4=0.005 Ohm  tau4=30 s  Rp5=0.005 Ohm  tau5=30 s  prm_fade=2  N_fade=200  AH_fade=56 hr*A  R1_fade=2.02 Ohm  V1_fade=10.35 V  i_specify=off  i_priority=None  i=0 A  i_nominal_specify=off  i_nominal_unit=A  i_nominal_value=1  v_specify=off  v_priority=None  v=0 V  v_nominal_specify=off  v_nominal_unit=V  v_nominal_value=1  charge_specify=on  charge_priority=High  charge="7  hr*A"  charge_nominal_specify=off  charge_nominal_unit=hr*A  charge_nominal_value=1  num_cycles_specify=off  num_cycles_priority=High  num_cycles=0  num_cycles_nominal_specify=off  num_cycles_nominal_unit=1  num_cycles_nominal_value=1  thermal_mass=30000 J/K  Tmeas=298.15 K  Vnom_T2=12 V  R1_T2=2.2 Ohm  V1_T2=11.4 V  R2_T2=2200 Ohm  Rp1_T2=0.005 Ohm  tau1_T2=30 s  Rp2_T2=0.005 Ohm  tau2_T2=30 s  Rp3_T2=0.005 Ohm  tau3_T2=30 s  Rp4_T2=0.005 Ohm  tau4_T2=30 s  Rp5_T2=0.005 Ohm  tau5_T2=30 s  Tmeas2=273.15 K  temperature_specify=off  temperature_priority=High  temperature=298.15 K  temperature_nominal_specify=off  temperature_nominal_unit=K  temperature_nominal_value=1
      settings: InternalSimscapePortConfiguration="{\"Bottom\":[],\"Left\":[{\"id\":\"p\",\"label\":\"+\",\"type\":\"foundation.electrical.electrical\"},{\"id\":\"q\",\"label\":\"q\",\"type\":\"output\"}],\"Right\":[{\"id\":\"n\",\"label\":\"-\",\"type\":\"foundation.electrical.electrical\"}],\"Top\":[]}"
  Coulomb pr Ah : Constant  Value=3600
  Current Sensor1 : fl_lib/Electrical/Electrical Sensors/Current Sensor
  PS-Simulink Converter : nesl_utility/PS-Simulink Converter  PhysicalDomain=network_engine_domain  SubClassName=ps_output  LeftPortType=input  RightPortType=output  PseudoPeriodic=off  Frequencies=[]  Unit=inherit  AffineConversion=off
  PS-Simulink Converter1 : nesl_utility/PS-Simulink Converter  PhysicalDomain=network_engine_domain  SubClassName=ps_output  LeftPortType=input  RightPortType=output  PseudoPeriodic=off  Frequencies=[]  Unit=inherit  AffineConversion=off
  PS-Simulink Converter3 : nesl_utility/PS-Simulink Converter  PhysicalDomain=network_engine_domain  SubClassName=ps_output  LeftPortType=input  RightPortType=output  PseudoPeriodic=off  Frequencies=[]  Unit=inherit  AffineConversion=off
  Percent SOC : Product  Inputs=*/
  Solver Configuration1 : nesl_utility/Solver Configuration  PhysicalDomain=network_engine_domain  SubClassName=solver  LeftPortType=input  RightPortType=generic  Tones=[]  Harmonics=[]  SimulateNoise=off  Profile=off  UseLocalSampling=off  EnableSwitchedLinearOptims=on  FrequencyDomain=off  UseCCode=off  RelTol=0.001  AbsTol=1e-06  MinStep=1e-09  ToWorkspace=off  RevertToSquareIcSolve=off  NumHomotopyIterations=100  PhasorMode=off  PhasorModeNumHarmonics=1  DoDC=off  ResidualTolerance=1e-09  UseLocalSolver=off  LocalSolverChoice=NE_BACKWARD_EULER_ADVANCER  LocalSolverSampleTime=0.001  DoFixedCost=off  MaxNonlinIter=3  MaxModeIter=2  LinearAlgebra=auto  EquationFormulation=NE_TIME_EF  DelaysMemoryBudget=1024  AutomaticFiltering=on  FilteringTimeConstant=0.001  PartitionStorageMethod=AS_NEEDED  PartitionMemoryBudget=1024  PartitionMethod=ROBUST
  Total Coulomb : Product  Inputs=**
  Voltage Sensor1 : fl_lib/Electrical/Electrical Sensors/Voltage Sensor
  Positiv pin : PMIOPort  Side=Right
  Negativ pin : PMIOPort  Port=2  Side=Right
  voltage : Outport
  current : Outport  Port=2
  SOC : Outport  Port=3
  wires:
  PS-Simulink Converter/1 -> current/1  "Current"
  PS-Simulink Converter1/1 -> voltage/1  "Voltage"
  Coulomb pr Ah/1 -> Total Coulomb/2
  Percent SOC/1 -> SOC/1  "State of Charge"
  PS-Simulink Converter3/1 -> Percent SOC/1  "Current Coulomb"
  Ah/1 -> Total Coulomb/1
  Total Coulomb/1 -> Percent SOC/2
  connections:
  Voltage Sensor1/RConn2 -- BlySyre/RConn1 -- Current Sensor1/RConn2
  BlySyre/LConn1 -- Positiv pin/RConn1 -- Voltage Sensor1/LConn1 -- Solver Configuration1/RConn1
  Current Sensor1/LConn1 -- Negativ pin/RConn1
  Current Sensor1/RConn1 -- PS-Simulink Converter/LConn1
  Voltage Sensor1/RConn1 -- PS-Simulink Converter1/LConn1
  BlySyre/LConn2 -- PS-Simulink Converter3/LConn1

== system Full_Charge/Opladning/Li-ion-3,6 ==
  Ah : Constant  Value=2.6
  Coulomb pr Ah : Constant  Value=3600
  Current Sensor1 : fl_lib/Electrical/Electrical Sensors/Current Sensor
  Li-ion 3,6V : ee_lib/Sources/Battery  Vnom=3.7 V  R1=0.07 Ohm  prm_AH=2  AH=2.6 hr*A  V1=3.2 V  AH1=0.52 hr*A  prm_R2=1  R2=5000 Ohm  prm_dyn=3  Rp1=0.0063 Ohm  tau1=111 s  Rp2=0.0043 Ohm  tau2=111 s  Rp3=0.005 Ohm  tau3=30 s  Rp4=0.005 Ohm  tau4=30 s  Rp5=0.005 Ohm  tau5=30 s  prm_fade=2  N_fade=300  AH_fade=2.08 hr*A  R1_fade=1.084 Ohm  V1_fade=0.208 V  i_specify=off  i_priority=None  i=0 A  i_nominal_specify=off  i_nominal_unit=A  i_nominal_value=1  v_specify=off  v_priority=None  v=0 V  v_nominal_specify=off  v_nominal_unit=V  v_nominal_value=1  charge_specify=on  charge_priority=High  charge=0.26 hr*A  charge_nominal_specify=off  charge_nominal_unit=hr*A  charge_nominal_value=1  num_cycles_specify=off  num_cycles_priority=High  num_cycles=0  num_cycles_nominal_specify=off  num_cycles_nominal_unit=1  num_cycles_nominal_value=1  thermal_mass=30000 J/K  Tmeas=298.15 K  Vnom_T2=12 V  R1_T2=2.2 Ohm  V1_T2=11.4 V  R2_T2=2200 Ohm  Rp1_T2=0.005 Ohm  tau1_T2=30 s  Rp2_T2=0.005 Ohm  tau2_T2=30 s  Rp3_T2=0.005 Ohm  tau3_T2=30 s  Rp4_T2=0.005 Ohm  tau4_T2=30 s  Rp5_T2=0.005 Ohm  tau5_T2=30 s  Tmeas2=273.15 K  temperature_specify=off  temperature_priority=High  temperature=298.15 K  temperature_nominal_specify=off  temperature_nominal_unit=K  temperature_nominal_value=1
      settings: InternalSimscapePortConfiguration="{\"Bottom\":[],\"Left\":[{\"id\":\"p\",\"label\":\"+\",\"type\":\"foundation.electrical.electrical\"},{\"id\":\"q\",\"label\":\"q\",\"type\":\"output\"}],\"Right\":[{\"id\":\"n\",\"label\":\"-\",\"type\":\"foundation.electrical.electrical\"}],\"Top\":[]}"
  PS-Simulink Converter : nesl_utility/PS-Simulink Converter  PhysicalDomain=network_engine_domain  SubClassName=ps_output  LeftPortType=input  RightPortType=output  PseudoPeriodic=off  Frequencies=[]  Unit=inherit  AffineConversion=off
  PS-Simulink Converter1 : nesl_utility/PS-Simulink Converter  PhysicalDomain=network_engine_domain  SubClassName=ps_output  LeftPortType=input  RightPortType=output  PseudoPeriodic=off  Frequencies=[]  Unit=inherit  AffineConversion=off
  PS-Simulink Converter2 : nesl_utility/PS-Simulink Converter  PhysicalDomain=network_engine_domain  SubClassName=ps_output  LeftPortType=input  RightPortType=output  PseudoPeriodic=off  Frequencies=[]  Unit=inherit  AffineConversion=off
  Percent SOC : Product  Inputs=*/
  Solver Configuration1 : nesl_utility/Solver Configuration  PhysicalDomain=network_engine_domain  SubClassName=solver  LeftPortType=input  RightPortType=generic  Tones=[]  Harmonics=[]  SimulateNoise=off  Profile=off  UseLocalSampling=off  EnableSwitchedLinearOptims=on  FrequencyDomain=off  UseCCode=off  RelTol=0.001  AbsTol=1e-06  MinStep=1e-09  ToWorkspace=off  RevertToSquareIcSolve=off  NumHomotopyIterations=100  PhasorMode=off  PhasorModeNumHarmonics=1  DoDC=off  ResidualTolerance=1e-09  UseLocalSolver=off  LocalSolverChoice=NE_BACKWARD_EULER_ADVANCER  LocalSolverSampleTime=0.001  DoFixedCost=off  MaxNonlinIter=3  MaxModeIter=2  LinearAlgebra=auto  EquationFormulation=NE_TIME_EF  DelaysMemoryBudget=1024  AutomaticFiltering=on  FilteringTimeConstant=0.001  PartitionStorageMethod=AS_NEEDED  PartitionMemoryBudget=1024  PartitionMethod=ROBUST
  Total Coulomb : Product  Inputs=**
  Voltage Sensor1 : fl_lib/Electrical/Electrical Sensors/Voltage Sensor
  Positiv pin : PMIOPort  Side=Right
  Negativ pin : PMIOPort  Port=2  Side=Right
  voltage : Outport
  current : Outport  Port=2
  SOC : Outport  Port=3
  wires:
  PS-Simulink Converter/1 -> current/1  "Current"
  PS-Simulink Converter1/1 -> voltage/1  "Voltage"
  Total Coulomb/1 -> Percent SOC/2
  Percent SOC/1 -> SOC/1  "State of Charge"
  Ah/1 -> Total Coulomb/1
  PS-Simulink Converter2/1 -> Percent SOC/1  "Current Coulomb"
  Coulomb pr Ah/1 -> Total Coulomb/2
  connections:
  Voltage Sensor1/RConn2 -- Li-ion 3,6V/RConn1 -- Current Sensor1/RConn2
  Li-ion 3,6V/LConn1 -- Positiv pin/RConn1 -- Voltage Sensor1/LConn1 -- Solver Configuration1/RConn1
  Current Sensor1/LConn1 -- Negativ pin/RConn1
  Current Sensor1/RConn1 -- PS-Simulink Converter/LConn1
  Voltage Sensor1/RConn1 -- PS-Simulink Converter1/LConn1
  Li-ion 3,6V/LConn2 -- PS-Simulink Converter2/LConn1

== system Full_Charge/Opladning/Li-ion-Batteri ==
  Ah : Constant  Value=12
  Coulomb pr Ah : Constant  Value=3600
  Current Sensor1 : fl_lib/Electrical/Electrical Sensors/Current Sensor
  Li-ion 12V : ee_lib/Sources/Battery  Vnom=12.8 V  R1=0.05 Ohm  prm_AH=2  AH=12 hr*A  V1=10.8 V  AH1=2 hr*A  prm_R2=1  R2=5000 Ohm  prm_dyn=3  Rp1=0.0063 Ohm  tau1=111 s  Rp2=0.0043 Ohm  tau2=111 s  Rp3=0.005 Ohm  tau3=30 s  Rp4=0.005 Ohm  tau4=30 s  Rp5=0.005 Ohm  tau5=30 s  prm_fade=2  N_fade=3000  AH_fade=10.2 hr*A  R1_fade=0.0575 Ohm  V1_fade=9.18 V  i_specify=off  i_priority=None  i=0 A  i_nominal_specify=off  i_nominal_unit=A  i_nominal_value=1  v_specify=off  v_priority=None  v=0 V  v_nominal_specify=off  v_nominal_unit=V  v_nominal_value=1  charge_specify=on  charge_priority=High  charge=1.2 hr*A  charge_nominal_specify=off  charge_nominal_unit=hr*A  charge_nominal_value=1  num_cycles_specify=off  num_cycles_priority=High  num_cycles=0  num_cycles_nominal_specify=off  num_cycles_nominal_unit=1  num_cycles_nominal_value=1  thermal_mass=30000 J/K  Tmeas=298.15 K  Vnom_T2=12 V  R1_T2=2.2 Ohm  V1_T2=11.4 V  R2_T2=2200 Ohm  Rp1_T2=0.005 Ohm  tau1_T2=30 s  Rp2_T2=0.005 Ohm  tau2_T2=30 s  Rp3_T2=0.005 Ohm  tau3_T2=30 s  Rp4_T2=0.005 Ohm  tau4_T2=30 s  Rp5_T2=0.005 Ohm  tau5_T2=30 s  Tmeas2=273.15 K  temperature_specify=off  temperature_priority=High  temperature=298.15 K  temperature_nominal_specify=off  temperature_nominal_unit=K  temperature_nominal_value=1
      settings: InternalSimscapePortConfiguration="{\"Bottom\":[],\"Left\":[{\"id\":\"p\",\"label\":\"+\",\"type\":\"foundation.electrical.electrical\"},{\"id\":\"q\",\"label\":\"q\",\"type\":\"output\"}],\"Right\":[{\"id\":\"n\",\"label\":\"-\",\"type\":\"foundation.electrical.electrical\"}],\"Top\":[]}"
  PS-Simulink Converter : nesl_utility/PS-Simulink Converter  PhysicalDomain=network_engine_domain  SubClassName=ps_output  LeftPortType=input  RightPortType=output  PseudoPeriodic=off  Frequencies=[]  Unit=inherit  AffineConversion=off
  PS-Simulink Converter1 : nesl_utility/PS-Simulink Converter  PhysicalDomain=network_engine_domain  SubClassName=ps_output  LeftPortType=input  RightPortType=output  PseudoPeriodic=off  Frequencies=[]  Unit=inherit  AffineConversion=off
  PS-Simulink Converter2 : nesl_utility/PS-Simulink Converter  PhysicalDomain=network_engine_domain  SubClassName=ps_output  LeftPortType=input  RightPortType=output  PseudoPeriodic=off  Frequencies=[]  Unit=inherit  AffineConversion=off
  Percent SOC : Product  Inputs=*/
  Solver Configuration1 : nesl_utility/Solver Configuration  PhysicalDomain=network_engine_domain  SubClassName=solver  LeftPortType=input  RightPortType=generic  Tones=[]  Harmonics=[]  SimulateNoise=off  Profile=off  UseLocalSampling=off  EnableSwitchedLinearOptims=on  FrequencyDomain=off  UseCCode=off  RelTol=0.001  AbsTol=1e-06  MinStep=1e-09  ToWorkspace=off  RevertToSquareIcSolve=off  NumHomotopyIterations=100  PhasorMode=off  PhasorModeNumHarmonics=1  DoDC=off  ResidualTolerance=1e-09  UseLocalSolver=off  LocalSolverChoice=NE_BACKWARD_EULER_ADVANCER  LocalSolverSampleTime=0.001  DoFixedCost=off  MaxNonlinIter=3  MaxModeIter=2  LinearAlgebra=auto  EquationFormulation=NE_TIME_EF  DelaysMemoryBudget=1024  AutomaticFiltering=on  FilteringTimeConstant=0.001  PartitionStorageMethod=AS_NEEDED  PartitionMemoryBudget=1024  PartitionMethod=ROBUST
  Total Coulomb : Product  Inputs=**
  Voltage Sensor1 : fl_lib/Electrical/Electrical Sensors/Voltage Sensor
  Positiv pin : PMIOPort  Side=Right
  Negativ pin : PMIOPort  Port=2  Side=Right
  voltage : Outport
  current : Outport  Port=2
  SOC : Outport  Port=3
  wires:
  PS-Simulink Converter/1 -> current/1  "Current"
  PS-Simulink Converter1/1 -> voltage/1  "Voltage"
  Percent SOC/1 -> SOC/1  "State of Charge"
  Coulomb pr Ah/1 -> Total Coulomb/2
  PS-Simulink Converter2/1 -> Percent SOC/1  "Current Coulomb"
  Ah/1 -> Total Coulomb/1
  Total Coulomb/1 -> Percent SOC/2
  connections:
  Voltage Sensor1/RConn2 -- Li-ion 12V/RConn1 -- Current Sensor1/RConn2
  Li-ion 12V/LConn1 -- Positiv pin/RConn1 -- Voltage Sensor1/LConn1 -- Solver Configuration1/RConn1
  Current Sensor1/LConn1 -- Negativ pin/RConn1
  Current Sensor1/RConn1 -- PS-Simulink Converter/LConn1
  Voltage Sensor1/RConn1 -- PS-Simulink Converter1/LConn1
  PS-Simulink Converter2/LConn1 -- Li-ion 12V/LConn2

== system Full_Charge/Opladning/NiMH ==
  note: Panasonic BK120AAHU
  Bus Selector : BusSelector  OutputSignals=Current (A),Voltage (V),SOC (%)
  Gain : Gain  Gain=1/100
  Ni-MH 1.2AH : electricdrivelib/Extra Sources/Battery  BatType=Nickel-Metal-Hydride  ShowTempParam=off  ThermalPreset=no  ShowAgeParam=off  NomV=1.22  NomQ=1.2  SOC=10  Batt_Tr=30  PresetModel=off  MaxQ=1.291  MinV=0.915  FullV=1.43  Dis_rate=0.240  R=0.017  Normal_OP=1.128  expZone="[1.27        0.24]"  current=[0.240 0.480 1.2]  Units=Time  Tci=20  NomT=20  T2=-30  MaxQ2=4.8  FullV2=7.1  Normal_OP2=5.655  expZone2="[6.58           1]"  Rca=0.6  ti=2000  Dp=0  Neq0=0  Tsim=1e6  Ta1=25  Qeol=5.4*0.9  Reol=0.013333*1.2  Char_age=[2.3478, 3]  Dis_age=[2.3478, 10]  N1=1500  N2=10500  N3=1000  N4=1400  Ta2=45  N5=950
  powergui : powerlib/powergui  Priority=1  SimulationMode=Continuous  SampleTime=50e-6  frequency=60  Iterations=50  frequencyindice=0  Pbase=100e6  ErrMax=1e-4  UnitsV=kV  UnitsW=MW  buscounter=0  FunctionMessages=off  echomessages=off  EnableUseOfTLC=off  CurrentSourceSwitches=off  DisableSnubberDevices=off  DisableRonSwitches=off  DisableVfSwitches=off  DisplayEquations=off  AutomaticDiscreteSolvers=off  SolverType=Tustin/Backward Euler (TBE)  Interpol=off  ExternalGateDelay=off  methode=off  Ts=100  x0status=blocks  SPID=on  SwTol=0  HookPort=off  NonlinearTolerance=1e-4  nMaxIteration=100  ContinueOnMaxIteration=off  RestoreLinks=warning  ResistiveCurrentMeasurement=off  Frange=[0:2:500]  Ylog=off  Xlog=on  ShowGrid=off  save=off  variable=ZData  structure=0  ZoomFFT=off  StartTime=0.0  cycles=1  DisplayStyle=1  fundamental=60  FreqAxis=off  MaxFrequency=1000  frequencyindicesteady=1  RmsSteady=1  display=off
  Positiv : PMIOPort  Side=Right
  Negativ : PMIOPort  Port=2  Side=Right
  VoltageLevel : Outport
  CurrentLevel : Outport  Port=2
  SOC : Outport  Port=3
  wires:
  Bus Selector/1 -> CurrentLevel/1  "<Current (A)>"
  Ni-MH 1.2AH/1 -> Bus Selector/1
  Bus Selector/2 -> VoltageLevel/1  "<Voltage (V)>"
  Bus Selector/3 -> Gain/1  "<SOC (%)>"
  Gain/1 -> SOC/1
  connections:
  Ni-MH 1.2AH/LConn1 -- Positiv/RConn1
  Ni-MH 1.2AH/LConn2 -- Negativ/RConn1
